simulink model "dat_dict_blocks_ex"  (R2022b)
settings: Solver=VariableStepAuto  StartTime=0.0  StopTime=10.0  RelTol=1e-3
values from neighbouring files (symbols this model uses):
  gain1 = 3.0    [data_dict_values_ex.sldd]
  gain2 = 5.0    [data_dict_values_ex.sldd]
  Num1 = 10.0    [data_dict_values_ex.sldd]
  Num2 = 20.0    [data_dict_values_ex.sldd]
  Num3 = 2.0    [data_dict_values_ex.sldd]
  Num4 = 50.0    [data_dict_values_ex.sldd]
settings Model: DataDictionary=data_dict_values_ex.sldd  Creator=Brigosha_Guest  LastModifiedBy=Brigosha_Guest

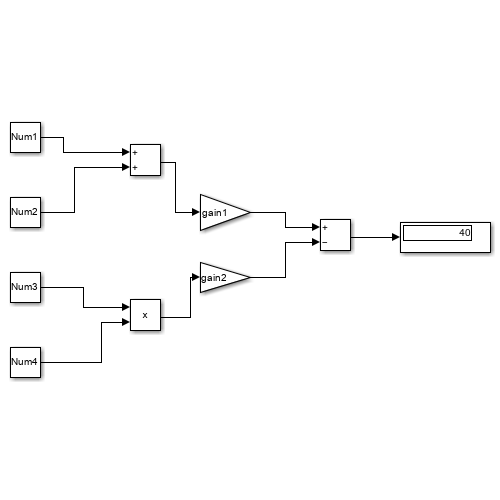
[thumbnail: Simulink's stored preview of the top-level diagram]
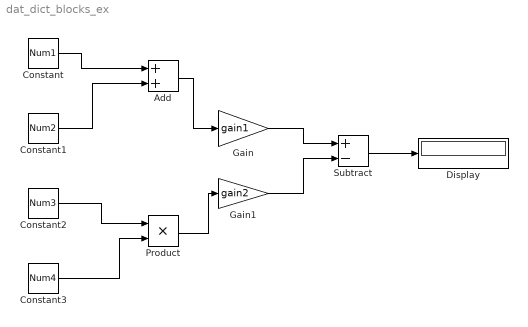
== system dat_dict_blocks_ex ==
  Add : Sum
  Constant : Constant  Value=Num1
  Constant1 : Constant  Value=Num2
  Constant2 : Constant  Value=Num3
  Constant3 : Constant  Value=Num4
  Display : Display
  Gain : Gain  Gain=gain1
  Gain1 : Gain  Gain=gain2
  Product : Product
  Subtract : Sum  Inputs=+-
  wires:
  Gain1/1 -> Subtract/2
  Constant1/1 -> Add/2
  Constant2/1 -> Product/1
  Constant3/1 -> Product/2
  Subtract/1 -> Display/1
  Product/1 -> Gain1/1
  Add/1 -> Gain/1
  Constant/1 -> Add/1
  Gain/1 -> Subtract/1
